simulink model "model"  (R2014a)
settings: Solver=ode3  StartTime=0.0  StopTime=10.0  FixedStep=0.01  RelTol=1e-3
values from neighbouring files (symbols this model uses):
  A = [0,1;0,-1.782000000000000]    [ModelValues.m]    (also in modelerwin.mat = [-2.02973141125  0.612067387973; -0.07490477511  -2.45796858; newpoles.m = A_old2-B*K)
  B = [0;-39.940000000000000]    [ModelValues.m]    (also in modelerwin.mat = [2.4327 6.1289])
  C = [1,0]    [ModelValues.m]    (also in modelerwin.mat = [7.8178 -7.0269])
  C2 = [1 0]    [modelerwin.mat]
  K = acker(A, B, K_poles)    [ModelValues.m]    (also in modelerwin.mat = [-0.19331137779 -0.170019320147]; newpoles.m = acker(A_old2,B,poles))
  L = acker(A', C', L_poles)    [ModelValues.m]    (also in modelerwin.mat = [0.677100111676 0.253473544958]; newpoles.m = acker(A',C',Lpoles)')
undefined symbols (not defined in the file or in its folder): A2
libraries: simulink x1
settings Model: Creator=Sander  LastModifiedBy=Erwin
settings DebuggingCC: UnderspecifiedInitializationDetection=Classic

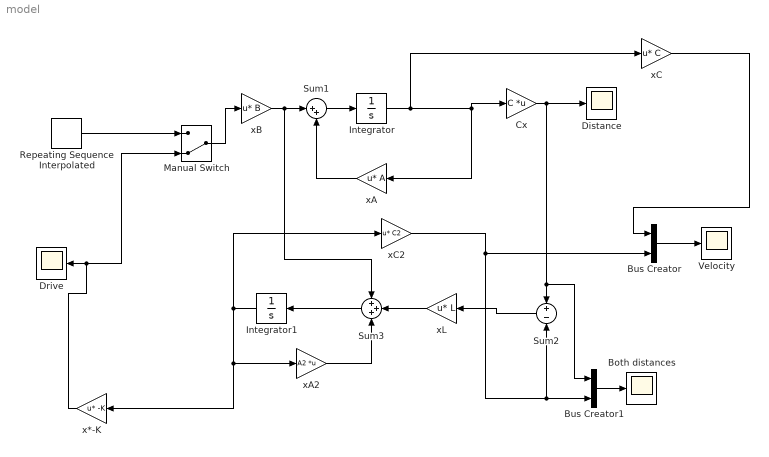
== system model ==
  Both distances : Scope
      settings: TimeRange=10  YMin=2.2872  YMax=2.2886  SaveName=ScopeData3
  Bus Creator : BusCreator  Inputs=2
  Bus Creator1 : BusCreator  Inputs=2
  Cx : Gain  Gain=C  Multiplication=Matrix(K*u)
  Distance : Scope
      settings: TimeRange=10  YMin=2.2872  YMax=2.2886
  Drive : Scope
      settings: TimeRange=10  YMin=-1e+61  YMax=0
  Integrator : Integrator  InitialCondition=[3;-3]
  Integrator1 : Integrator  InitialCondition=[3;-3]
  Manual Switch : ManualSwitch  CurrentSetting=0
  Repeating Sequence Interpolated : simulink/Sources/Repeating Sequence Interpolated  OutValues=[0 0.3 0.1 0.4 0.2 0.1].'  TimeValues=[0 0.1 0.5 0.6 0.8 1].'  LookUpMeth=Interpolation-Use End Values  tsamp=0.01  OutMin=[]  OutMax=[]  OutDataTypeStr=double  OutputDataTypeScalingMode=double  OutDataType=fixdt(0,8)  OutScaling=2^-10
  Sum1 : Sum  Inputs=|++
  Sum2 : Sum  Inputs=+|-
  Sum3 : Sum  Inputs=+++
  Velocity : Scope
      settings: TimeRange=10  YMin=2.2872  YMax=2.2886  SaveName=ScopeData2
  x*-K : Gain  Gain=-K  Multiplication=Matrix(u*K)
  xA : Gain  Gain=A  Multiplication=Matrix(u*K)
  xA2 : Gain  Gain=A2  Multiplication=Matrix(K*u)
  xB : Gain  Gain=B  Multiplication=Matrix(u*K)
  xC : Gain  Gain=C  Multiplication=Matrix(u*K)
  xC2 : Gain  Gain=C2  Multiplication=Matrix(u*K)
  xL : Gain  Gain=L  Multiplication=Matrix(u*K)
  wires:
  Sum1/1 -> Integrator/1
  xA/1 -> Sum1/2
  xB/1 -> Sum3/1, Sum1/1
  Sum2/1 -> xL/1
  Sum3/1 -> Integrator1/1
  xA2/1 -> Sum3/3
  Integrator/1 -> xC/1, Cx/1, xA/1
  Bus Creator/1 -> Velocity/1
  xC/1 -> Bus Creator/1
  xC2/1 -> Bus Creator1/2, Sum2/2, Bus Creator/2
  xL/1 -> Sum3/2
  Bus Creator1/1 -> Both distances/1
  Cx/1 -> Bus Creator1/1, Sum2/1, Distance/1
  Repeating Sequence Interpolated/1 -> Manual Switch/1
  Integrator1/1 -> xC2/1, x*-K/1, xA2/1
  x*-K/1 -> Manual Switch/2, Drive/1
  Manual Switch/1 -> xB/1
